simulink model "Coastdown"  (R2019a)
settings: Solver=FixedStepAuto  StartTime=0.0  StopTime=600  FixedStep=Ts  MaxStep=Ts  RelTol=1e-3
PreLoadFcn:
  | Ts = Ts;
values from neighbouring files (symbols this model uses):
  I_initial = v_desired/(R_bx)    (= 0)    [parameters.m]
  Jb = (m_b)*((R_bxb)^2)    (= 41.86125)    [parameters.m]
  Jx = (m_x)*((R_bx)^2)    (= 29.64574716)    [parameters.m]
  m_x = 159    [parameters.m]
  R_bx = 0.4318    [parameters.m]
  R_bxb = 0.305    [parameters.m]
libraries: powerlib x9, simulink x2
settings Model: SimulationMode=accelerator  Creator=Phuc  LastModifiedBy=Dinh Ngoc Quy
settings SolverCC: AlgebraicLoopSolver=LineSearch
settings DataIOCC: ReturnWorkspaceOutputs=off
settings DebuggingCC: AlgebraicLoopMsg=none  ArithmeticOperatorsInVariantConditions=warning
settings SFSimCC: SimUseLocalCustomCode=off
settings RTWCC: RTWUseLocalCustomCode=off

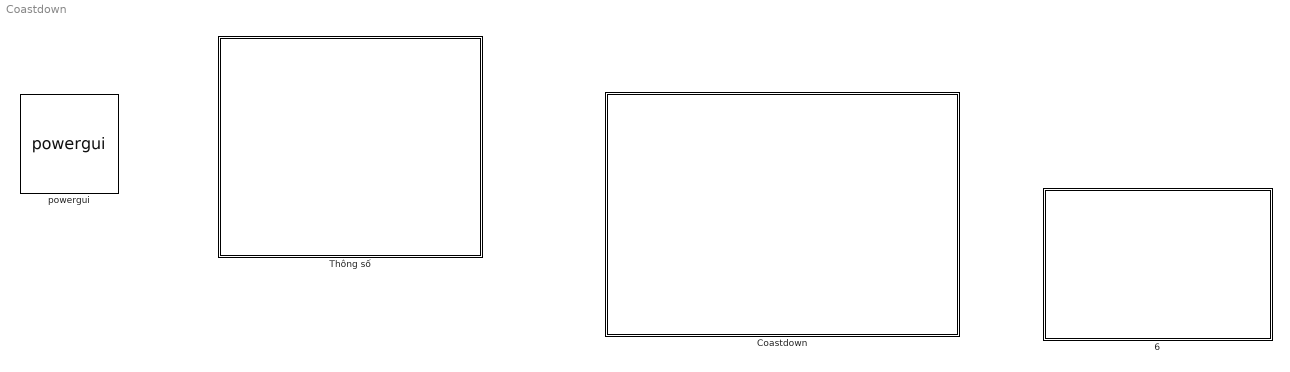
== system Coastdown ==
  6 : Subsystem
      mask Display:
      | image('motorelec.jpg')
      | port_label('input',1,'w (rad/s)')
  Coastdown : Subsystem
      mask Display:
      | IconInfo = autosharedicon('autolibvehdyncdt', gcb, 4);
      | 
      |     image(IconInfo.image, IconInfo.position);
      | 
      |     for i = 1:numel(IconInfo.lconn)
      |         port_label('lconn', i, IconInfo.lconn{i})
      |     end
      | 
      |     for j = 1:numel(IconInfo.rconn)
      |         port_label('rconn', j, IconInfo.rconn{j})
      |     end
      | 
      |     for k = 1:numel(IconInfo.input)
      |         port_label('input', k, IconInfo.input{k})
      |     end
      | 
      |     for m = 1:numel(IconInfo.output)
      |         port_label('output', m, IconInfo.output{m})
      |     end
  Thông số : Subsystem  VariantControl=Variant1
  powergui : powerlib/powergui  SimulationMode=Discrete  SampleTime=Ts  frequency=60  Iterations=50  frequencyindice=50  Pbase=100e6  ErrMax=1e-4  UnitsV=kV  UnitsW=MW  buscounter=0  FunctionMessages=off  echomessages=off  EnableUseOfTLC=off  CurrentSourceSwitches=off  DisableSnubberDevices=off  DisableRonSwitches=off  DisableVfSwitches=off  DisplayEquations=off  AutomaticDiscreteSolvers=off  SolverType=Tustin/Backward Euler (TBE)  Interpol=off  ExternalGateDelay=off  methode=off  Ts=100  x0status=blocks  SPID=off  SwTol=0  HookPort=off  NonlinearTolerance=0  nMaxIteration=15  ContinueOnMaxIteration=off  RestoreLinks=warning  ResistiveCurrentMeasurement=off  Frange=[0:2:500]  Ylog=off  Xlog=on  ShowGrid=off  save=off  variable=ZData  structure=0  ZoomFFT=on  StartTime=0.0  cycles=1  DisplayStyle=1  fundamental=60  FreqAxis=off  MaxFrequency=1000  frequencyindicesteady=1  RmsSteady=1  display=off
      settings: SourceProductName=Simscape Electrical

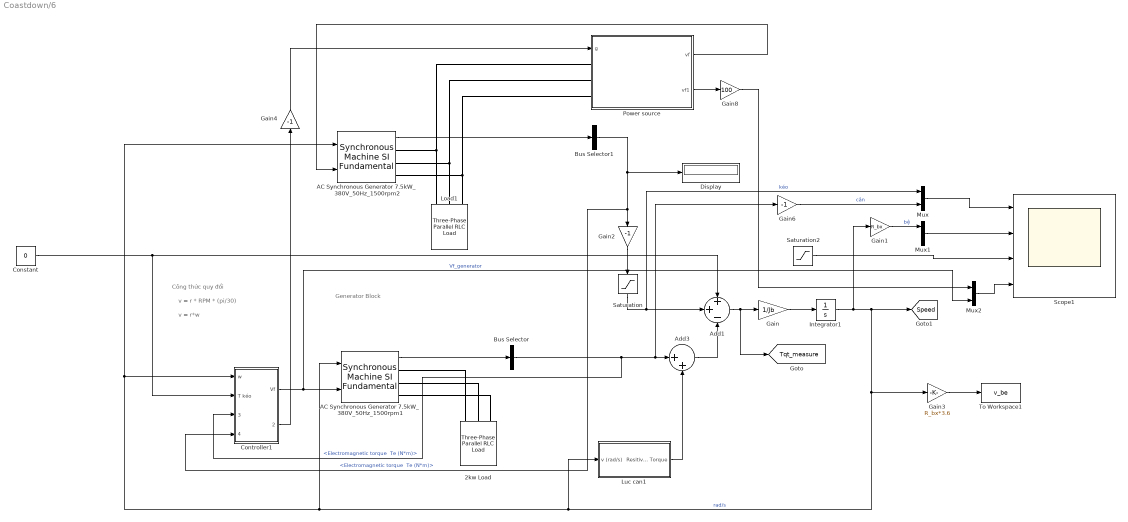
== system Coastdown/6 ==
  note: v = r*w
  note: v = r * RPM * (pi/30)
  note: Công thức quy đổi
  note: Generator Block
  2kw Load : powerlib/Elements/Three-Phase Parallel RLC Load  LConnTagsString=A|B|C  Configuration=Y (grounded)  NominalVoltage=220  Vabc=[1e3 1e3 1e3]  Vabcp=[1e3 1e3 1e3]  NominalFrequency=50  UnbalancedPower=off  ActivePower=5000  InductivePower=0  CapacitivePower=0  Pabc=[10e3 9e3 11e3]  QLabc=[100 90 110]  QCabc=[100 90 110]  Pabcp=[10e3 9e3 11e3]  QLabcp=[100 90 110]  QCabcp=[100 90 110]  Measurements=None  LoadType=constant Z
      settings: SourceProductName=Simscape Electrical
  AC Synchronous Generator 7.5kW_380V_50Hz_1500rpm1 : powerlib/Machines/Synchronous Machine SI Fundamental  PresetModel=No  MechanicalLoad=Speed w  ShowDetailedParameters=on  RotorType=Salient-pole  Units=SI fundamental parameters  MeasurementBus=off  NominalParameters=[7500 380 50 4]  Stator=[1.62 0.004527 0.1086 0.05175]  Field=[1.208 0.01132]  Dampers2=[ 0.0664, 1.387e-3, 0.0292, 6.896e-4, 7.907e-3, 2.477e-3]  Dampers1=[3.142 0.007334 4.772 0.01015]  Mechanical=[0.0923 0.009 2]  PolePairs=2  InitialConditions="[ 0  0  0  0  0  0  0  0 0]"  SetSaturation=off  Saturation=[695.64,774.7,917.5,1001.6,1082.2,1175.9,1293.6,1430.2,1583.7;9660,10623,12243,13063,13757,14437,15180,15890,16567]  DisplayVfd=off  LoadFlowParameters=[1,0,0,0,0]  TsPowergui=0  TsBlock=-1  IterativeModel=Trapezoidal non iterative  IterativeDiscreteModel=Trapezoidal non iterative  BusType=swing  Pref=0  Qref=0  Qmin=-inf  Qmax=inf  PLF=0  QLF=0
      settings: SourceProductName=Simscape Electrical  SourceProductBaseCode=PS
  AC Synchronous Generator 7.5kW_380V_50Hz_1500rpm2 : powerlib/Machines/Synchronous Machine SI Fundamental  PresetModel=No  MechanicalLoad=Speed w  ShowDetailedParameters=on  RotorType=Salient-pole  Units=SI fundamental parameters  MeasurementBus=off  NominalParameters=[7500 380 50 4]  Stator=[1.62 0.004527 0.1086 0.05175]  Field=[1.208 0.01132]  Dampers2=[ 0.0664, 1.387e-3, 0.0292, 6.896e-4, 7.907e-3, 2.477e-3]  Dampers1=[3.142 0.007334 4.772 0.01015]  Mechanical=[0.0923 0.009 2]  PolePairs=2  InitialConditions="[ 0  0  0  0  0  0  0  0 0]"  SetSaturation=off  Saturation=[695.64,774.7,917.5,1001.6,1082.2,1175.9,1293.6,1430.2,1583.7;9660,10623,12243,13063,13757,14437,15180,15890,16567]  DisplayVfd=off  LoadFlowParameters=[1,0,0,0,0]  TsPowergui=0  TsBlock=-1  IterativeModel=Trapezoidal non iterative  IterativeDiscreteModel=Trapezoidal non iterative  BusType=swing  Pref=0  Qref=0  Qmin=-inf  Qmax=inf  PLF=0  QLF=0
      settings: SourceProductName=Simscape Electrical  SourceProductBaseCode=PS
  Add1 : Sum  Inputs=++-
  Add3 : Sum  Inputs=|++
  Bus Selector : BusSelector  OutputSignals="Mechanical.Electromagnetic torque  Te (N*m)"
  Bus Selector1 : BusSelector  OutputSignals="Mechanical.Electromagnetic torque  Te (N*m)"
  Constant : Constant  Value=0
  Controller1 : Subsystem
  Display : Display
  Gain : Gain  Gain=1/Jb
  Gain1 : Gain  Gain=R_bx
  Gain2 : Gain  Gain=-1
  Gain3 : Gain  Gain=R_bx*3.6
  Gain4 : Gain  Gain=-1
  Gain6 : Gain  Gain=-1
  Gain8 : Gain  Gain=100
  Integrator1 : Integrator  InitialCondition=I_initial  LimitOutput=on  LowerSaturationLimit=0  ContinuousStateAttributes='velocity'
  Load1 : powerlib/Elements/Three-Phase Parallel RLC Load  LConnTagsString=A|B|C  Configuration=Y (grounded)  NominalVoltage=220  Vabc=[1e3 1e3 1e3]  Vabcp=[1e3 1e3 1e3]  NominalFrequency=50  UnbalancedPower=off  ActivePower=7500  InductivePower=0  CapacitivePower=0  Pabc=[10e3 9e3 11e3]  QLabc=[100 90 110]  QCabc=[100 90 110]  Pabcp=[10e3 9e3 11e3]  QLabcp=[100 90 110]  QCabcp=[100 90 110]  Measurements=None  LoadType=constant Z
      settings: SourceProductName=Simscape Electrical
  Luc can1 : Subsystem
  Mux : Mux  Inputs=2
  Mux1 : Mux  Inputs=2
  Mux2 : Mux  Inputs=2
  Power source : Subsystem
  Saturation : Saturate  UpperLimit=inf  LowerLimit=0
  Saturation2 : Saturate  UpperLimit=inf  LowerLimit=0
  Scope1 : Scope  NumInputPorts=4
  To Workspace1 : ToWorkspace  VariableName=v_be  SaveFormat=Structure With Time  SampleTime=-1
  tag scope: Speed=global, Tqt_measure=global
  wires:
  Saturation2/1 -> Scope1/3
  Gain4/1 -> Power source/1(g)
  Gain8/1 -> Mux2/1
  Power source/2(vf1) -> Gain8/1
  Mux2/1 -> Scope1/4
  Mux1/1 -> Scope1/2
  Mux/1 -> Scope1/1
  Gain1/1 -> Mux1/1  "bệ"
  Power source/1(vf) -> AC Synchronous Generator 7.5kW_380V_50Hz_1500rpm2/2
  Controller1/1(Vf) -> AC Synchronous Generator 7.5kW_380V_50Hz_1500rpm1/2, Mux2/2  "Vf_generator"
  AC Synchronous Generator 7.5kW_380V_50Hz_1500rpm1/1 -> Bus Selector/1
  Gain/1 -> Integrator1/1
  Bus Selector/1 -> Controller1/3(T_measured), Add3/1, Gain6/1  "<Electromagnetic torque  Te (N*m)>"
  Add1/1 -> Gain/1, [Tqt_measure]
  Luc can1/1(Resitive Torque) -> Add3/2
  Add3/1 -> Add1/3
  AC Synchronous Generator 7.5kW_380V_50Hz_1500rpm2/1 -> Bus Selector1/1
  Bus Selector1/1 -> Controller1/4(T_motor), Gain2/1, Display/1  "<Electromagnetic torque  Te (N*m)>"
  Gain2/1 -> Saturation/1
  Integrator1/1 -> Gain3/1, Luc can1/1(v (rad/s)), AC Synchronous Generator 7.5kW_380V_50Hz_1500rpm2/1, Controller1/1(w), AC Synchronous Generator 7.5kW_380V_50Hz_1500rpm1/1, [Speed], Gain1/1  "rad/s"
  Saturation/1 -> Mux/1, Add1/2  "kéo"
  Gain6/1 -> Mux/2  "cản"
  Controller1/2(Vf_motor) -> Gain4/1
  Constant/1 -> Controller1/2(T kéo), Add1/1
  Gain3/1 -> To Workspace1/1
  connections:
  AC Synchronous Generator 7.5kW_380V_50Hz_1500rpm1/RConn1 -- 2kw Load/LConn1
  AC Synchronous Generator 7.5kW_380V_50Hz_1500rpm1/RConn3 -- 2kw Load/LConn3
  AC Synchronous Generator 7.5kW_380V_50Hz_1500rpm1/RConn2 -- 2kw Load/LConn2
  Load1/LConn1 -- Power source/LConn1 -- AC Synchronous Generator 7.5kW_380V_50Hz_1500rpm2/RConn1
  Load1/LConn2 -- Power source/LConn2 -- AC Synchronous Generator 7.5kW_380V_50Hz_1500rpm2/RConn2
  Load1/LConn3 -- Power source/LConn3 -- AC Synchronous Generator 7.5kW_380V_50Hz_1500rpm2/RConn3

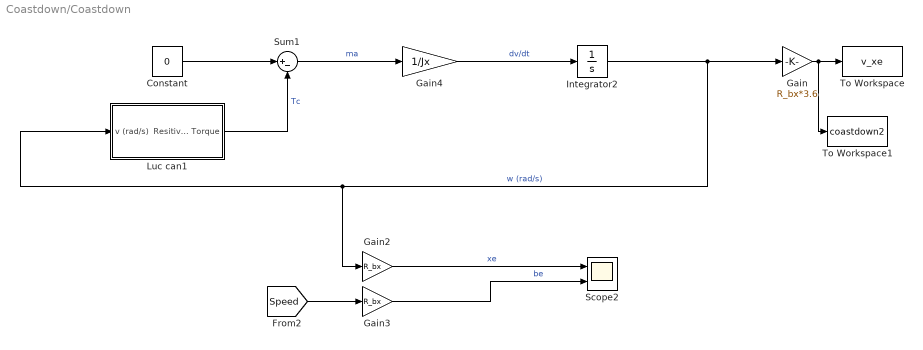
== system Coastdown/Coastdown ==
  Constant : Constant  Value=0
  Gain : Gain  Gain=R_bx*3.6
  Gain2 : Gain  Gain=R_bx
  Gain3 : Gain  Gain=R_bx
  Gain4 : Gain  Gain=1/Jx
  Integrator2 : Integrator  InitialCondition=I_initial  LimitOutput=on  LowerSaturationLimit=0  ContinuousStateAttributes='velocity'
  Luc can1 : Subsystem
  Scope2 : Scope  NumInputPorts=2
  Sum1 : Sum  Inputs=|+-
  To Workspace : ToWorkspace  VariableName=v_xe  SaveFormat=Structure With Time  SampleTime=-1
  To Workspace1 : ToWorkspace  VariableName=coastdown2  SaveFormat=Timeseries  SampleTime=1
  wires:
  Gain3/1 -> Scope2/2  "be"
  [Speed] -> Gain3/1
  Luc can1/1(Resitive Torque) -> Sum1/2  "Tc"
  Sum1/1 -> Gain4/1  "ma"
  Gain4/1 -> Integrator2/1  "dv/dt"
  Constant/1 -> Sum1/1
  Gain2/1 -> Scope2/1  "xe"
  Gain/1 -> To Workspace1/1, To Workspace/1
  Integrator2/1 -> Luc can1/1(v (rad/s)), Gain2/1, Gain/1  "w (rad/s)"

== system Coastdown/Thông số ==
  note: Thông số
  note: c_d : Hệ số cản khí động của xe
  note: p : Mật độ kk tại điều kiện thường
  note: c_d : Hệ số cản khí động
  note: Area : Diện tích cản chính diện của xe (m^2)
  note: alpha : Gốc leo dốc
  note: f : Hệ số cản lăn của đường
  note: i_d: tỉ số bộ truyền đai
  note: Công thức quy đổi
  note: v_desired: tốc độ mong muốn (m/s)
  note: v = r * RPM * (pi/30)
  note: g : trọng lượng
  note: a, b, c: hệ số cản ma sát trên bệ
  note: R_bx: bán kính bánh xe trên bệ
  note: v = r*w
  note: m_x: khối lượng xe (kg)

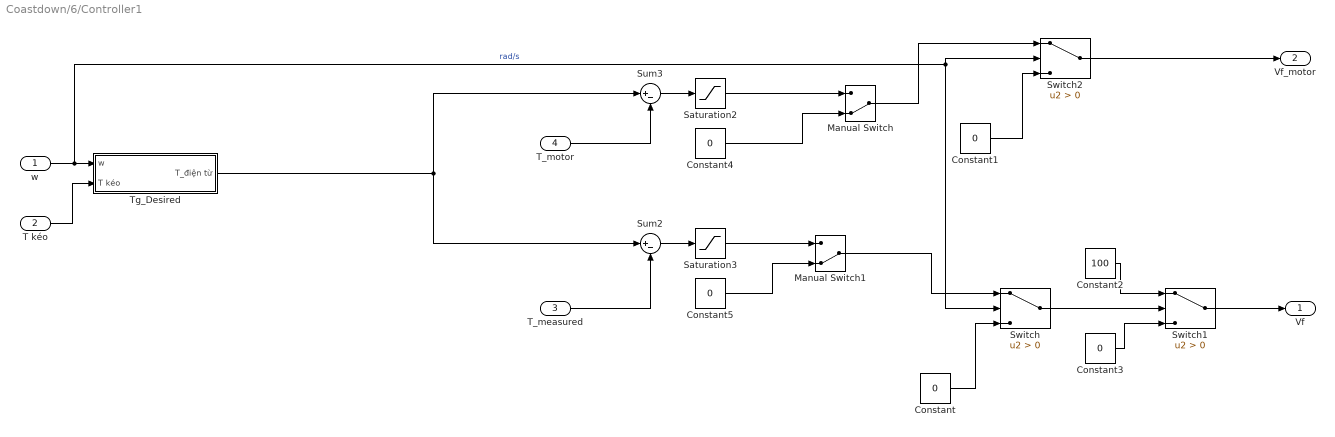
== system Coastdown/6/Controller1 ==
  w : Inport
  T kéo : Inport  Port=2
  T_measured : Inport  Port=3
  T_motor : Inport  Port=4
  Constant{,1,3..5} (5 alike) : Constant  Value=0
  Constant2 : Constant  Value=100
  Manual Switch : ManualSwitch  CurrentSetting=0
  Manual Switch1 : ManualSwitch  CurrentSetting=0
  Saturation2 : Saturate  UpperLimit=0  LowerLimit=-inf
  Saturation3 : Saturate  UpperLimit=inf  LowerLimit=0
  Sum2 : Sum  Inputs=|+-
  Sum3 : Sum  Inputs=|+-
  Switch : Switch  Criteria=u2 > Threshold
  Switch1 : Switch  Criteria=u2 > Threshold
  Switch2 : Switch  Criteria=u2 > Threshold
  Tg_Desired : Subsystem
  Vf : Outport
  Vf_motor : Outport  Port=2
  wires:
  Switch/1 -> Switch1/2
  Constant/1 -> Switch/3
  w/1 -> Switch/2, Switch2/2, Tg_Desired/1(w)  "rad/s"
  T kéo/1 -> Tg_Desired/2(T kéo)
  Constant2/1 -> Switch1/1
  Constant3/1 -> Switch1/3
  Switch1/1 -> Vf/1
  Sum2/1 -> Saturation3/1
  T_measured/1 -> Sum2/2
  T_motor/1 -> Sum3/2
  Switch2/1 -> Vf_motor/1
  Sum3/1 -> Saturation2/1
  Constant1/1 -> Switch2/3
  Tg_Desired/1(T_điện từ) -> Sum2/1, Sum3/1
  Constant4/1 -> Manual Switch/2
  Saturation2/1 -> Manual Switch/1
  Manual Switch/1 -> Switch2/1
  Constant5/1 -> Manual Switch1/2
  Saturation3/1 -> Manual Switch1/1
  Manual Switch1/1 -> Switch/1

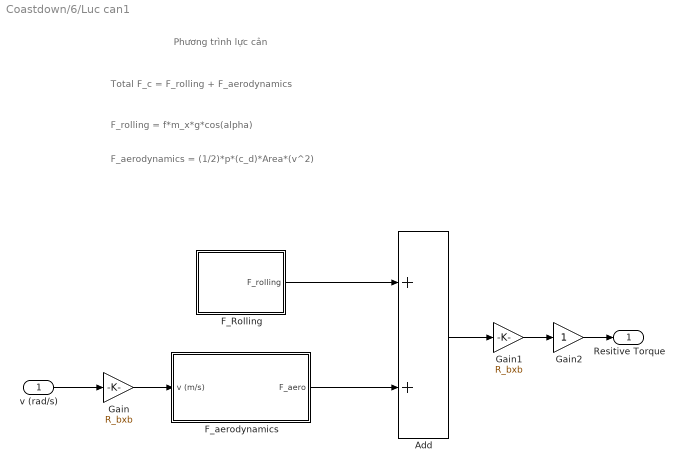
== system Coastdown/6/Luc can1 ==
  note: Phương trình lực cản
  note: F_aerodynamics = (1/2)*p*(c_d)*Area*(v^2)
  note: F_rolling = f*m_x*g*cos(alpha)
  note: Total F_c = F_rolling + F_aerodynamics
  v (rad/s) : Inport
  Add : Sum
  F_Rolling : Subsystem
  F_aerodynamics : Subsystem
  Gain : Gain  Gain=R_bxb
  Gain1 : Gain  Gain=R_bxb
  Gain2 : Gain
  Resitive Torque : Outport
  wires:
  Gain/1 -> F_aerodynamics/1(v (m/s))
  Add/1 -> Gain1/1
  v (rad/s)/1 -> Gain/1
  F_aerodynamics/1(F_aero) -> Add/2
  Gain1/1 -> Gain2/1
  Gain2/1 -> Resitive Torque/1
  F_Rolling/1(F_rolling) -> Add/1

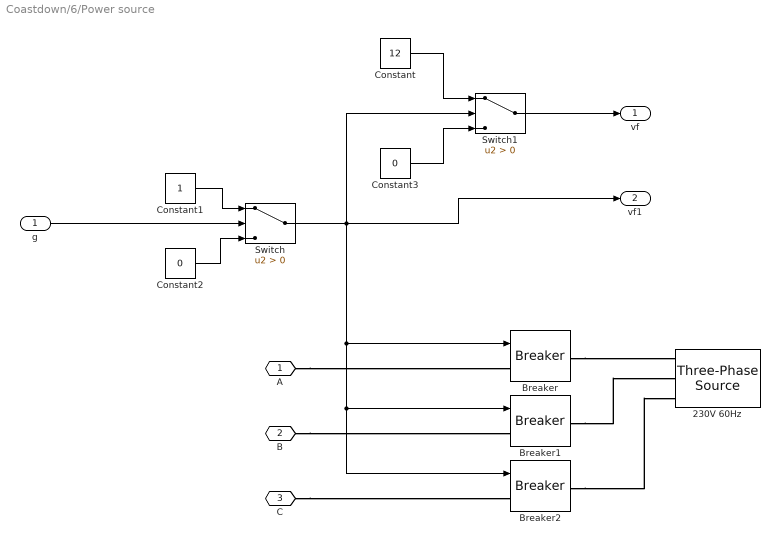
== system Coastdown/6/Power source ==
  g : Inport
  230V 60Hz : powerlib/Electrical Sources/Three-Phase Source  InternalConnection=Yg  VoltagePhases=off  Voltage=220  PhaseAngle=0  Voltage_phases=[25e3 25e3 25e3]/sqrt(3)  PhaseAngles_phases=[0 -120 +120]  Frequency=50  NonIdealSource=on  SpecifyImpedance=off  Resistance=0.0002  Inductance=0.05e-3  ShortCircuitLevel=100e6  BaseVoltage=380  XRratio=7  BusType=swing  Pref=0  Qref=0  Prefabc=[10e3, 10e3, 10e3]  Qrefabc=[0, 0, 0]  Qmin=-inf  Qmax=inf
      settings: SourceProductName=Simscape Electrical
  Breaker : powerlib/Elements/Breaker  InitialState=1  SwitchingTimes="[1/60  5/60]"  External=on  BreakerResistance=0.01  SnubberResistance=1e6  SnubberCapacitance=inf  Measurements=None  MoreParameters=on  NoBreakLoop=off
      settings: SourceProductName=Simscape Electrical
  Breaker1 : powerlib/Elements/Breaker  InitialState=1  SwitchingTimes="[1/60  5/60]"  External=on  BreakerResistance=0.01  SnubberResistance=1e6  SnubberCapacitance=inf  Measurements=None  MoreParameters=on  NoBreakLoop=off
      settings: SourceProductName=Simscape Electrical
  Breaker2 : powerlib/Elements/Breaker  InitialState=1  SwitchingTimes="[1/60  5/60]"  External=on  BreakerResistance=0.01  SnubberResistance=1e6  SnubberCapacitance=inf  Measurements=None  MoreParameters=on  NoBreakLoop=off
      settings: SourceProductName=Simscape Electrical
  Constant : Constant  Value=12
  Constant1 : Constant
  Constant2 : Constant  Value=0
  Constant3 : Constant  Value=0
  Switch : Switch  Criteria=u2 > Threshold
  Switch1 : Switch  Criteria=u2 > Threshold
  A : PMIOPort  Side=Left
  B : PMIOPort  Port=2  Side=Left
  C : PMIOPort  Port=3  Side=Left
  vf : Outport
  vf1 : Outport  Port=2
  wires:
  Switch/1 -> Switch1/2, Breaker2/1, Breaker1/1, Breaker/1, vf1/1
  Constant1/1 -> Switch/1
  Constant2/1 -> Switch/3
  g/1 -> Switch/2
  Constant/1 -> Switch1/1
  Constant3/1 -> Switch1/3
  Switch1/1 -> vf/1
  connections:
  Breaker2/RConn1 -- 230V 60Hz/RConn3
  Breaker/RConn1 -- 230V 60Hz/RConn1
  Breaker1/RConn1 -- 230V 60Hz/RConn2
  A/RConn1 -- Breaker/LConn1
  C/RConn1 -- Breaker2/LConn1
  B/RConn1 -- Breaker1/LConn1

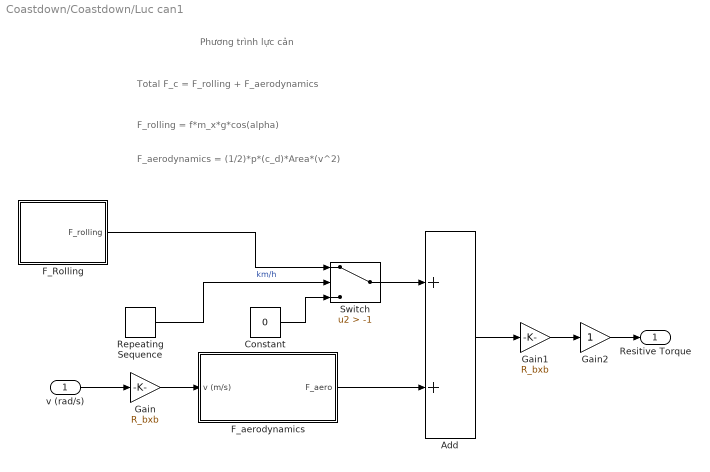
== system Coastdown/Coastdown/Luc can1 ==
  note: Phương trình lực cản
  note: F_aerodynamics = (1/2)*p*(c_d)*Area*(v^2)
  note: F_rolling = f*m_x*g*cos(alpha)
  note: Total F_c = F_rolling + F_aerodynamics
  v (rad/s) : Inport
  Add : Sum
  Constant : Constant  Value=0
  F_Rolling : Subsystem
  F_aerodynamics : Subsystem
  Gain : Gain  Gain=R_bxb
  Gain1 : Gain  Gain=R_bxb
  Gain2 : Gain
  Repeating Sequence : simulink/Sources/Repeating Sequence  rep_seq_t=DriveCycle_time  rep_seq_y=DriveCycle_speed
  Switch : Switch  Criteria=u2 > Threshold  Threshold=-1
  Resitive Torque : Outport
  wires:
  Gain/1 -> F_aerodynamics/1(v (m/s))
  Add/1 -> Gain1/1
  v (rad/s)/1 -> Gain/1
  F_aerodynamics/1(F_aero) -> Add/2
  Repeating Sequence/1 -> Switch/2  "km/h"
  Constant/1 -> Switch/3
  F_Rolling/1(F_rolling) -> Switch/1
  Switch/1 -> Add/1
  Gain1/1 -> Gain2/1
  Gain2/1 -> Resitive Torque/1

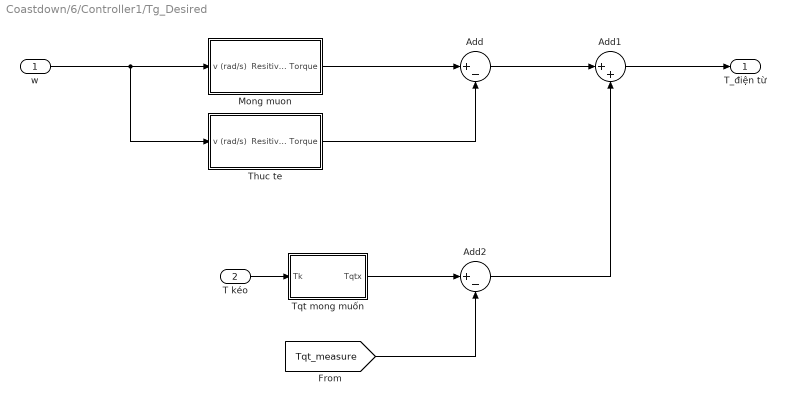
== system Coastdown/6/Controller1/Tg_Desired ==
  w : Inport
  T kéo : Inport  Port=2
  Add : Sum  Inputs=|+-
  Add1 : Sum  Inputs=|++
  Add2 : Sum  Inputs=|+-
  Mong muon : Subsystem
  Thuc te : Subsystem
  Tqt mong muốn : Subsystem
  T_điện từ : Outport
  wires:
  w/1 -> Mong muon/1(v (rad/s)), Thuc te/1(v (rad/s))
  [Tqt_measure] -> Add2/2
  Tqt mong muốn/1(Tqtx) -> Add2/1
  Thuc te/1(Resitive Torque) -> Add/2
  Add/1 -> Add1/1
  Add2/1 -> Add1/2
  T kéo/1 -> Tqt mong muốn/1(Tk)
  Add1/1 -> T_điện từ/1
  Mong muon/1(Resitive Torque) -> Add/1

== system Coastdown/6/Luc can1/F_Rolling ==
  Constant : Constant  Value=0.018
  Constant1 : Constant  Value=m_x
  Constant2 : Constant  Value=9.81
  Constant3 : Constant  Value=0
  Cos : Trigonometry  Operator=cos
  Product1 : Product  Inputs=4
  F_rolling : Outport
  wires:
  Constant2/1 -> Product1/3
  Constant3/1 -> Cos/1
  Product1/1 -> F_rolling/1
  Constant1/1 -> Product1/2
  Cos/1 -> Product1/4
  Constant/1 -> Product1/1

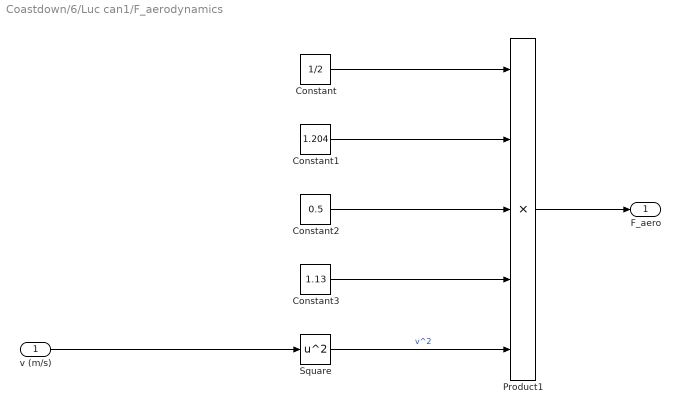
== system Coastdown/6/Luc can1/F_aerodynamics ==
  v (m/s) : Inport
  Constant : Constant  Value=1/2
  Constant1 : Constant  Value=1.204
  Constant2 : Constant  Value=0.5
  Constant3 : Constant  Value=1.13
  Product1 : Product  Inputs=5
  Square : Math  Operator=square  RndMeth=Zero  SaturateOnIntegerOverflow=on
  F_aero : Outport
  wires:
  v (m/s)/1 -> Square/1
  Constant/1 -> Product1/1
  Constant3/1 -> Product1/4
  Constant1/1 -> Product1/2
  Constant2/1 -> Product1/3
  Square/1 -> Product1/5  "v^2"
  Product1/1 -> F_aero/1

== system Coastdown/Coastdown/Luc can1/F_Rolling ==
  Constant : Constant  Value=0.018
  Constant1 : Constant  Value=m_x
  Constant2 : Constant  Value=9.81
  Constant3 : Constant  Value=0
  Cos : Trigonometry  Operator=cos
  Product1 : Product  Inputs=4
  F_rolling : Outport
  wires:
  Constant2/1 -> Product1/3
  Constant3/1 -> Cos/1
  Product1/1 -> F_rolling/1
  Constant1/1 -> Product1/2
  Cos/1 -> Product1/4
  Constant/1 -> Product1/1

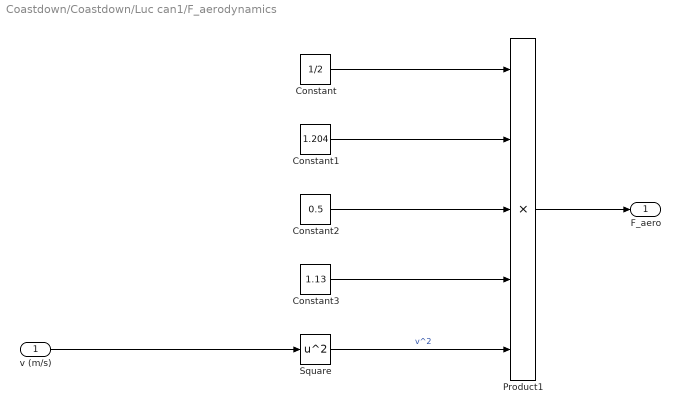
== system Coastdown/Coastdown/Luc can1/F_aerodynamics ==
  v (m/s) : Inport
  Constant : Constant  Value=1/2
  Constant1 : Constant  Value=1.204
  Constant2 : Constant  Value=0.5
  Constant3 : Constant  Value=1.13
  Product1 : Product  Inputs=5
  Square : Math  Operator=square  RndMeth=Zero  SaturateOnIntegerOverflow=on
  F_aero : Outport
  wires:
  v (m/s)/1 -> Square/1
  Constant/1 -> Product1/1
  Constant3/1 -> Product1/4
  Constant1/1 -> Product1/2
  Constant2/1 -> Product1/3
  Square/1 -> Product1/5  "v^2"
  Product1/1 -> F_aero/1

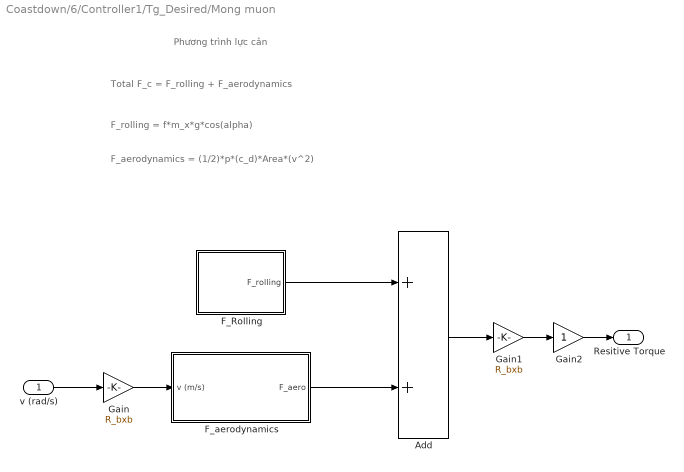
== system Coastdown/6/Controller1/Tg_Desired/Mong muon ==
  note: Phương trình lực cản
  note: F_aerodynamics = (1/2)*p*(c_d)*Area*(v^2)
  note: F_rolling = f*m_x*g*cos(alpha)
  note: Total F_c = F_rolling + F_aerodynamics
  v (rad/s) : Inport
  Add : Sum
  F_Rolling : Subsystem
  F_aerodynamics : Subsystem
  Gain : Gain  Gain=R_bxb
  Gain1 : Gain  Gain=R_bxb
  Gain2 : Gain
  Resitive Torque : Outport
  wires:
  Gain/1 -> F_aerodynamics/1(v (m/s))
  Add/1 -> Gain1/1
  v (rad/s)/1 -> Gain/1
  F_aerodynamics/1(F_aero) -> Add/2
  F_Rolling/1(F_rolling) -> Add/1
  Gain1/1 -> Gain2/1
  Gain2/1 -> Resitive Torque/1

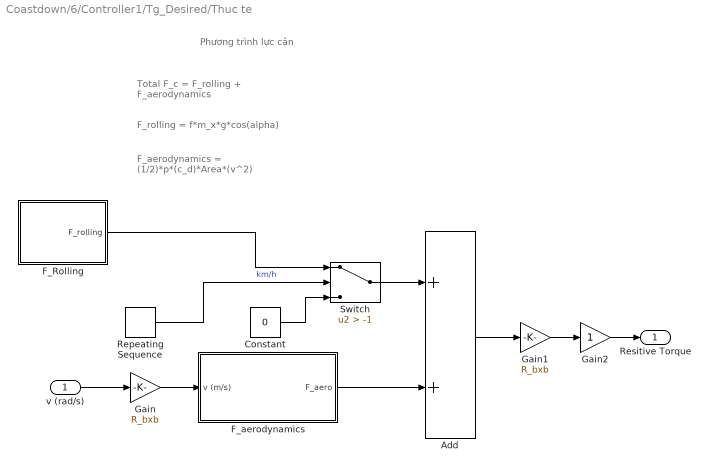
== system Coastdown/6/Controller1/Tg_Desired/Thuc te ==
  note: Phương trình lực cản
  note: F_aerodynamics = (1/2)*p*(c_d)*Area*(v^2)
  note: F_rolling = f*m_x*g*cos(alpha)
  note: Total F_c = F_rolling + F_aerodynamics
  v (rad/s) : Inport
  Add : Sum
  Constant : Constant  Value=0
  F_Rolling : Subsystem
  F_aerodynamics : Subsystem
  Gain : Gain  Gain=R_bxb
  Gain1 : Gain  Gain=R_bxb
  Gain2 : Gain
  Repeating Sequence : simulink/Sources/Repeating Sequence  rep_seq_t=DriveCycle_time  rep_seq_y=DriveCycle_speed
  Switch : Switch  Criteria=u2 > Threshold  Threshold=-1
  Resitive Torque : Outport
  wires:
  Gain/1 -> F_aerodynamics/1(v (m/s))
  Add/1 -> Gain1/1
  v (rad/s)/1 -> Gain/1
  F_aerodynamics/1(F_aero) -> Add/2
  Repeating Sequence/1 -> Switch/2  "km/h"
  Constant/1 -> Switch/3
  F_Rolling/1(F_rolling) -> Switch/1
  Switch/1 -> Add/1
  Gain1/1 -> Gain2/1
  Gain2/1 -> Resitive Torque/1

== system Coastdown/6/Controller1/Tg_Desired/Tqt mong muốn ==
  Tk : Inport
  Gain1 : Gain  Gain=1/Jx
  Integrator1 : Integrator  InitialCondition=I_initial  LimitOutput=on  LowerSaturationLimit=0  ContinuousStateAttributes='velocity'
  Luc can1 : Subsystem
  Sum1 : Sum  Inputs=|+-
  Tqtx : Outport
  wires:
  Gain1/1 -> Integrator1/1  "dv/dt"
  Tk/1 -> Sum1/1
  Sum1/1 -> Gain1/1, Tqtx/1  "ma"
  Integrator1/1 -> Luc can1/1(v (rad/s))  "v(rad/s)"
  Luc can1/1(Resitive Torque) -> Sum1/2  "Tc"

== system Coastdown/6/Controller1/Tg_Desired/Mong muon/F_Rolling ==
  Constant : Constant  Value=0.018
  Constant1 : Constant  Value=m_x
  Constant2 : Constant  Value=9.81
  Constant3 : Constant  Value=0
  Cos : Trigonometry  Operator=cos
  Product1 : Product  Inputs=4
  F_rolling : Outport
  wires:
  Constant2/1 -> Product1/3
  Constant3/1 -> Cos/1
  Product1/1 -> F_rolling/1
  Constant1/1 -> Product1/2
  Cos/1 -> Product1/4
  Constant/1 -> Product1/1

== system Coastdown/6/Controller1/Tg_Desired/Mong muon/F_aerodynamics ==
  v (m/s) : Inport
  Constant : Constant  Value=1/2
  Constant1 : Constant  Value=1.204
  Constant2 : Constant  Value=0.5
  Constant3 : Constant  Value=1.13
  Product1 : Product  Inputs=5
  Square : Math  Operator=square  RndMeth=Zero  SaturateOnIntegerOverflow=on
  F_aero : Outport
  wires:
  v (m/s)/1 -> Square/1
  Constant/1 -> Product1/1
  Constant3/1 -> Product1/4
  Constant1/1 -> Product1/2
  Constant2/1 -> Product1/3
  Square/1 -> Product1/5  "v^2"
  Product1/1 -> F_aero/1

== system Coastdown/6/Controller1/Tg_Desired/Thuc te/F_Rolling ==
  Constant : Constant  Value=0.018
  Constant1 : Constant  Value=m_x
  Constant2 : Constant  Value=9.81
  Constant3 : Constant  Value=0
  Cos : Trigonometry  Operator=cos
  Product1 : Product  Inputs=4
  F_rolling : Outport
  wires:
  Constant2/1 -> Product1/3
  Constant3/1 -> Cos/1
  Product1/1 -> F_rolling/1
  Constant1/1 -> Product1/2
  Cos/1 -> Product1/4
  Constant/1 -> Product1/1

== system Coastdown/6/Controller1/Tg_Desired/Thuc te/F_aerodynamics ==
  v (m/s) : Inport
  Constant : Constant  Value=1/2
  Constant1 : Constant  Value=1.204
  Constant2 : Constant  Value=0.5
  Constant3 : Constant  Value=1.13
  Product1 : Product  Inputs=5
  Square : Math  Operator=square  RndMeth=Zero  SaturateOnIntegerOverflow=on
  F_aero : Outport
  wires:
  v (m/s)/1 -> Square/1
  Constant/1 -> Product1/1
  Constant3/1 -> Product1/4
  Constant1/1 -> Product1/2
  Constant2/1 -> Product1/3
  Square/1 -> Product1/5  "v^2"
  Product1/1 -> F_aero/1

== system Coastdown/6/Controller1/Tg_Desired/Tqt mong muốn/Luc can1 ==
  note: Phương trình lực cản
  note: F_aerodynamics = (1/2)*p*(c_d)*Area*(v^2)
  note: F_rolling = f*m_x*g*cos(alpha)
  note: Total F_c = F_rolling + F_aerodynamics
  v (rad/s) : Inport
  Add : Sum
  F_Rolling : Subsystem
  F_aerodynamics : Subsystem
  Gain : Gain  Gain=R_bxb
  Gain1 : Gain  Gain=R_bxb
  Gain2 : Gain
  Resitive Torque : Outport
  wires:
  Gain/1 -> F_aerodynamics/1(v (m/s))
  Add/1 -> Gain1/1
  v (rad/s)/1 -> Gain/1
  F_aerodynamics/1(F_aero) -> Add/2
  F_Rolling/1(F_rolling) -> Add/1
  Gain1/1 -> Gain2/1
  Gain2/1 -> Resitive Torque/1

== system Coastdown/6/Controller1/Tg_Desired/Tqt mong muốn/Luc can1/F_Rolling ==
  Constant : Constant  Value=0.018
  Constant1 : Constant  Value=m_x
  Constant2 : Constant  Value=9.81
  Constant3 : Constant  Value=0
  Cos : Trigonometry  Operator=cos
  Product1 : Product  Inputs=4
  F_rolling : Outport
  wires:
  Constant2/1 -> Product1/3
  Constant3/1 -> Cos/1
  Product1/1 -> F_rolling/1
  Constant1/1 -> Product1/2
  Cos/1 -> Product1/4
  Constant/1 -> Product1/1

== system Coastdown/6/Controller1/Tg_Desired/Tqt mong muốn/Luc can1/F_aerodynamics ==
  v (m/s) : Inport
  Constant : Constant  Value=1/2
  Constant1 : Constant  Value=1.204
  Constant2 : Constant  Value=0.5
  Constant3 : Constant  Value=1.13
  Product1 : Product  Inputs=5
  Square : Math  Operator=square  RndMeth=Zero  SaturateOnIntegerOverflow=on
  F_aero : Outport
  wires:
  v (m/s)/1 -> Square/1
  Constant/1 -> Product1/1
  Constant3/1 -> Product1/4
  Constant1/1 -> Product1/2
  Constant2/1 -> Product1/3
  Square/1 -> Product1/5  "v^2"
  Product1/1 -> F_aero/1
